simulink model "HDD_MinJerk"  (R2017a)
settings: Solver=VariableStepAuto  StartTime=0.0  StopTime=0.02  FixedStep=1e-4  RelTol=1e-3
undefined symbols (not defined in the file or in its folder): Gp, Gv
libraries: cstblocks x4
settings Model: Creator=peter  LastModifiedBy=capn

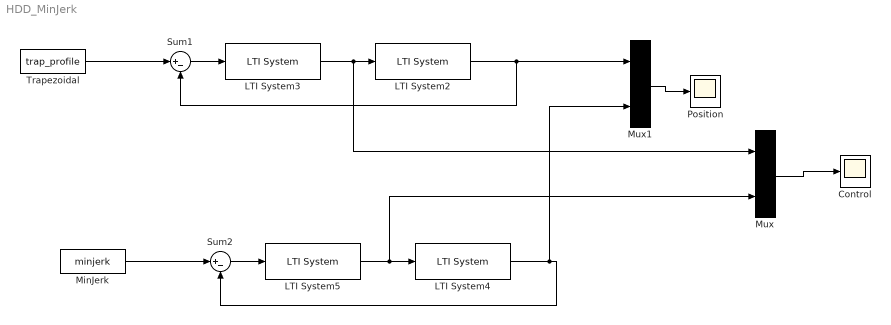
== system HDD_MinJerk ==
  Control : Scope
  LTI System2 : cstblocks/LTI System  sys=[Gv Gp]  IC=[]
  LTI System3 : cstblocks/LTI System  sys=Kinf  IC=[]
  LTI System4 : cstblocks/LTI System  sys=[Gv Gp]  IC=[]
  LTI System5 : cstblocks/LTI System  sys=Kinf  IC=[]
  MinJerk : FromWorkspace  VariableName=minjerk  SampleTime=0  OutputAfterFinalValue=Holding final value
  Mux : Mux  Inputs=2
  Mux1 : Mux  Inputs=2
  Position : Scope
  Sum1 : Sum  Inputs=|+-
  Sum2 : Sum  Inputs=|+-
  Trapezoidal : FromWorkspace  VariableName=trap_profile  SampleTime=0  OutputAfterFinalValue=Holding final value
  wires:
  LTI System2/1 -> Mux1/1, Sum1/2
  Trapezoidal/1 -> Sum1/1
  Sum1/1 -> LTI System3/1
  LTI System3/1 -> Mux/1, LTI System2/1
  LTI System4/1 -> Mux1/2, Sum2/2
  MinJerk/1 -> Sum2/1
  Sum2/1 -> LTI System5/1
  Mux/1 -> Control/1
  Mux1/1 -> Position/1
  LTI System5/1 -> Mux/2, LTI System4/1
